simulink model "IEEE_5Bus_system_load_flow"  (R2025a)
settings: Solver=VariableStepAuto  StartTime=0.0  StopTime=10.0  RelTol=1e-3
libraries: spsThreePhasePISectionLineLib x7, spsThreePhaseVIMeasurementLib x5, spsLoadFlowBusLib x5, spsThreePhaseSeriesRLCLoadLib x4, spsThreePhaseSourceLib x2, spsThreePhaseFaultLib x1, sps_lib x1
settings Model: Creator=Hafizur Rahman  LastModifiedBy=pavan
settings RTWCC: GPUComputeCapability=3.5

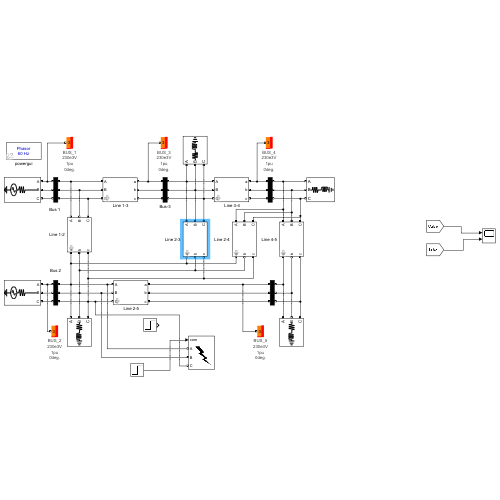
[thumbnail: Simulink's stored preview of the top-level diagram]
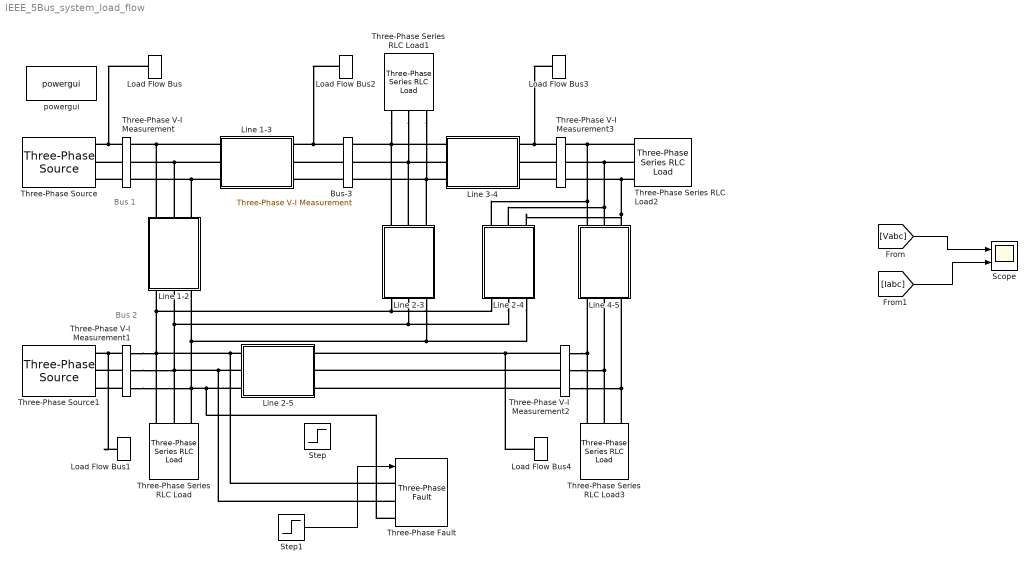
== system IEEE_5Bus_system_load_flow ==
  note: Bus 2
  note: Bus 1
  " Line 1-2" : Subsystem  mask{F=60, SB=100e6, V=230e3, R=0.02, X=0.06, B=0.06}
      mask prompts: F "Frequency"; SB "Base power"; V "Nominal Voltage"; R "Resistance(pu)"; X "Reactance(pu)"; B "Line Charging"
  " Line 1-3" : Subsystem  mask{F=60, SB=100e6, V=230e3, R=0.08, X=0.24, B=0.05}
      mask prompts: F "Frequency"; SB "Base power"; V "Nominal Voltage"; R "Resistance(pu)"; X "Reactance(pu)"; B "Line Charging"
  " Line 2-3" : Subsystem  mask{F=60, SB=100e6, V=230e3, R=0.06, X=0.18, B=0.04}
      mask prompts: F "Frequency"; SB "Base power"; V "Nominal Voltage"; R "Resistance(pu)"; X "Reactance(pu)"; B "Line Charging"
  " Line 2-4" : Subsystem  mask{F=60, SB=100e6, V=230e3, R=0.06, X=0.18, B=0.04}
      mask prompts: F "Frequency"; SB "Base power"; V "Nominal Voltage"; R "Resistance(pu)"; X "Reactance(pu)"; B "Line Charging"
  " Line 2-5" : Subsystem  mask{F=60, SB=100e6, V=230e3, R=0.04, X=0.12, B=0.03}
      mask prompts: F "Frequency"; SB "Base power"; V "Nominal Voltage"; R "Resistance(pu)"; X "Reactance(pu)"; B "Line Charging"
  " Line 3-4" : Subsystem  mask{F=60, SB=100e6, V=230e3, R=0.01, X=0.03, B=0.02}
      mask prompts: F "Frequency"; SB "Base power"; V "Nominal Voltage"; R "Resistance(pu)"; X "Reactance(pu)"; B "Line Charging"
  " Line 4-5" : Subsystem  mask{F=60, SB=100e6, V=230e3, R=0.08, X=0.24, B=0.05}
      mask prompts: F "Frequency"; SB "Base power"; V "Nominal Voltage"; R "Resistance(pu)"; X "Reactance(pu)"; B "Line Charging"
  Bus-3 : spsThreePhaseVIMeasurementLib/Three-Phase V-I Measurement  VoltageMeasurement=no  SetLabelV=off  LabelV=Vabc  Vpu=off  VpuLL=off  CurrentMeasurement=no  SetLabelI=off  LabelI=Iabc  Ipu=off  Pbase=100e6  Vbase=500e3  OutputType=Complex  PhasorSimulation=on  PSBequivalent=0
  Load Flow Bus : spsLoadFlowBusLib/Load Flow Bus  LConnTagsString=a  Phases=single  Connectors=on one side  ID=BUS_1  Vbase=230e3  Vref=1.06  Vangle=0  VLF=1  VLFb=1  VLFc=1  angleLF=0  angleLFb=0  angleLFc=0
  Load Flow Bus1 : spsLoadFlowBusLib/Load Flow Bus  LConnTagsString=a  Phases=single  Connectors=on one side  ID=BUS_2  Vbase=230e3  Vref=1  Vangle=0  VLF=1  VLFb=1  VLFc=1  angleLF=0  angleLFb=0  angleLFc=0
  Load Flow Bus2 : spsLoadFlowBusLib/Load Flow Bus  LConnTagsString=a  Phases=single  Connectors=on one side  ID=BUS_3  Vbase=230e3  Vref=1  Vangle=0  VLF=1  VLFb=1  VLFc=1  angleLF=0  angleLFb=0  angleLFc=0
  Load Flow Bus3 : spsLoadFlowBusLib/Load Flow Bus  LConnTagsString=a  Phases=single  Connectors=on one side  ID=BUS_4  Vbase=230e3  Vref=1  Vangle=0  VLF=1  VLFb=1  VLFc=1  angleLF=0  angleLFb=0  angleLFc=0
  Load Flow Bus4 : spsLoadFlowBusLib/Load Flow Bus  LConnTagsString=a  Phases=single  Connectors=on one side  ID=BUS_5  Vbase=230e3  Vref=1  Vangle=0  VLF=1  VLFb=1  VLFc=1  angleLF=0  angleLFb=0  angleLFc=0
  Scope : Scope  NumInputPorts=2
      settings: ActiveDisplayYMinimum=324868.26374899194  ActiveDisplayYMaximum=325037.04001697229
  Step : Step  SampleTime=0
  Step1 : Step  Time=5  SampleTime=0
  Three-Phase Series RLC Load : spsThreePhaseSeriesRLCLoadLib/Three-Phase Series RLC Load  LConnTagsString=A|B|C  Configuration=Y (grounded)  NominalVoltage=230e3  Vabc=[1e3 1e3 1e3]  Vabcp=[1e3 1e3 1e3]  NominalFrequency=60  UnbalancedPower=off  ActivePower=20e6  InductivePower=10e6  CapacitivePower=0  Pabc=[10e3 9e3 11e3]  QLabc=[100 90 110]  QCabc=[100 90 110]  Pabcp=[10e3 9e3 11e3]  QLabcp=[100 90 110]  QCabcp=[100 90 110]  Measurements=None  LoadType=constant PQ
  Three-Phase Series RLC Load1 : spsThreePhaseSeriesRLCLoadLib/Three-Phase Series RLC Load  LConnTagsString=A|B|C  Configuration=Y (grounded)  NominalVoltage=230e3  Vabc=[1e3 1e3 1e3]  Vabcp=[1e3 1e3 1e3]  NominalFrequency=60  UnbalancedPower=off  ActivePower=45e6  InductivePower=15e6  CapacitivePower=0  Pabc=[10e3 9e3 11e3]  QLabc=[100 90 110]  QCabc=[100 90 110]  Pabcp=[10e3 9e3 11e3]  QLabcp=[100 90 110]  QCabcp=[100 90 110]  Measurements=None  LoadType=constant PQ
  Three-Phase Series RLC Load2 : spsThreePhaseSeriesRLCLoadLib/Three-Phase Series RLC Load  LConnTagsString=A|B|C  Configuration=Y (grounded)  NominalVoltage=230e3  Vabc=[1e3 1e3 1e3]  Vabcp=[1e3 1e3 1e3]  NominalFrequency=60  UnbalancedPower=off  ActivePower=40e6  InductivePower=5e6  CapacitivePower=0  Pabc=[10e3 9e3 11e3]  QLabc=[100 90 110]  QCabc=[100 90 110]  Pabcp=[10e3 9e3 11e3]  QLabcp=[100 90 110]  QCabcp=[100 90 110]  Measurements=None  LoadType=constant PQ
  Three-Phase Series RLC Load3 : spsThreePhaseSeriesRLCLoadLib/Three-Phase Series RLC Load  LConnTagsString=A|B|C  Configuration=Y (grounded)  NominalVoltage=230e3  Vabc=[1e3 1e3 1e3]  Vabcp=[1e3 1e3 1e3]  NominalFrequency=60  UnbalancedPower=off  ActivePower=60e6  InductivePower=10e6  CapacitivePower=0  Pabc=[10e3 9e3 11e3]  QLabc=[100 90 110]  QCabc=[100 90 110]  Pabcp=[10e3 9e3 11e3]  QLabcp=[100 90 110]  QCabcp=[100 90 110]  Measurements=None  LoadType=constant PQ
  Three-Phase V-I Measurement : spsThreePhaseVIMeasurementLib/Three-Phase V-I Measurement  VoltageMeasurement=no  SetLabelV=off  LabelV=Vabc  Vpu=off  VpuLL=off  CurrentMeasurement=no  SetLabelI=off  LabelI=Iabc  Ipu=off  Pbase=100e6  Vbase=500e3  OutputType=Complex  PhasorSimulation=on  PSBequivalent=0
  Three-Phase V-I Measurement1 : spsThreePhaseVIMeasurementLib/Three-Phase V-I Measurement  VoltageMeasurement=phase-to-phase  SetLabelV=on  LabelV=Vabc  Vpu=off  VpuLL=off  CurrentMeasurement=yes  SetLabelI=on  LabelI=Iabc  Ipu=off  Pbase=100e6  Vbase=500e3  OutputType=Magnitude  PhasorSimulation=on  PSBequivalent=0
  Three-Phase V-I Measurement2 : spsThreePhaseVIMeasurementLib/Three-Phase V-I Measurement  VoltageMeasurement=no  SetLabelV=off  LabelV=Vabc  Vpu=off  VpuLL=off  CurrentMeasurement=no  SetLabelI=off  LabelI=Iabc  Ipu=off  Pbase=100e6  Vbase=500e3  OutputType=Complex  PhasorSimulation=on  PSBequivalent=0
  Three-Phase V-I Measurement3 : spsThreePhaseVIMeasurementLib/Three-Phase V-I Measurement  VoltageMeasurement=no  SetLabelV=off  LabelV=Vabc  Vpu=off  VpuLL=off  CurrentMeasurement=no  SetLabelI=off  LabelI=Iabc  Ipu=off  Pbase=100e6  Vbase=500e3  OutputType=Complex  PhasorSimulation=on  PSBequivalent=0
  Three-Phase Fault : spsThreePhaseFaultLib/Three-Phase Fault  InitialStates=0  FaultA=on  FaultB=on  FaultC=on  GroundFault=on  SwitchTimes="[1/60  5/60]"  External=on  SwitchStatus=NaN  FaultResistance=0.001  GroundResistance=0.01  SnubberResistance=1e6  SnubberCapacitance=inf  Measurements=None
  Three-Phase Source : spsThreePhaseSourceLib/Three-Phase Source  InternalConnection=Yg  VoltagePhases=off  Voltage=1.06*230e3  PhaseAngle=0  Voltage_phases=[25e3 25e3 25e3]/sqrt(3)  PhaseAngles_phases=[0 -120 +120]  Frequency=60  NonIdealSource=on  SpecifyImpedance=off  Resistance=1e-6  Inductance=0  ShortCircuitLevel=100e6  BaseVoltage=230e3  XRratio=7  BusType=swing  Pref=10e3  Qref=0  Prefabc=[10e3, 10e3, 10e3]  Qrefabc=[0, 0, 0]  Qmin=-inf  Qmax=inf
  Three-Phase Source1 : spsThreePhaseSourceLib/Three-Phase Source  InternalConnection=Yg  VoltagePhases=off  Voltage=230e3  PhaseAngle=0  Voltage_phases=[25e3 25e3 25e3]/sqrt(3)  PhaseAngles_phases=[0 -120 +120]  Frequency=60  NonIdealSource=on  SpecifyImpedance=off  Resistance=1e-6  Inductance=0  ShortCircuitLevel=100e6  BaseVoltage=230e3  XRratio=7  BusType=PV  Pref=40e6  Qref=0  Prefabc=[10e3, 10e3, 10e3]  Qrefabc=[0, 0, 0]  Qmin=-300e6  Qmax=300e6
  powergui : sps_lib/powergui  Priority=1  SimulationMode=Phasor  SampleTime=50e-6  frequency=60  Iterations=50  frequencyindice=60  Pbase=100e6  ErrMax=1e-4  UnitsV=kV  UnitsW=MW  buscounter=0  FunctionMessages=off  echomessages=off  EnableUseOfTLC=off  CurrentSourceSwitches=off  DisableSnubberDevices=off  DisableRonSwitches=off  DisableVfSwitches=off  DisplayEquations=off  AutomaticDiscreteSolvers=off  SolverType=Tustin/Backward Euler (TBE)  Interpol=off  ExternalGateDelay=off  methode=off  Ts=100  x0status=blocks  SPID=on  SwTol=0  HookPort=off  NonlinearTolerance=1e-4  nMaxIteration=100  ContinueOnMaxIteration=off  RestoreLinks=warning  ResistiveCurrentMeasurement=off  Frange=[0:2:500]  Ylog=off  Xlog=on  ShowGrid=off  save=off  variable=ZData  structure=0  ZoomFFT=off  StartTime=0.0  cycles=1  DisplayStyle=1  fundamental=60  FreqAxis=off  MaxFrequency=1000  frequencyindicesteady=1  RmsSteady=1  display=off
  wires:
  Step1/1 -> Three-Phase Fault/1
  [Vabc] -> Scope/1
  [Iabc] -> Scope/2
  connections:
  Three-Phase V-I Measurement/LConn2 -- Three-Phase Source/RConn2
  Three-Phase V-I Measurement/LConn1 -- Load Flow Bus/LConn1 -- Three-Phase Source/RConn1
  Three-Phase V-I Measurement/LConn3 -- Three-Phase Source/RConn3
  " Line 1-3"/LConn1 -- " Line 1-2"/LConn1 -- Three-Phase V-I Measurement/RConn1
  " Line 1-3"/LConn2 -- " Line 1-2"/LConn2 -- Three-Phase V-I Measurement/RConn2
  " Line 1-3"/LConn3 -- " Line 1-2"/LConn3 -- Three-Phase V-I Measurement/RConn3
  Three-Phase V-I Measurement1/LConn1 -- Load Flow Bus1/LConn1 -- Three-Phase Source1/RConn1
  Three-Phase V-I Measurement1/LConn2 -- Three-Phase Source1/RConn2
  Three-Phase V-I Measurement1/LConn3 -- Three-Phase Source1/RConn3
  Three-Phase V-I Measurement1/RConn1 -- Three-Phase Fault/LConn1 -- " Line 2-5"/LConn1 -- Three-Phase Series RLC Load/LConn1 -- " Line 2-4"/RConn1 -- " Line 2-3"/RConn1 -- " Line 1-2"/RConn1
  Three-Phase V-I Measurement1/RConn2 -- Three-Phase Fault/LConn2 -- " Line 2-5"/LConn2 -- Three-Phase Series RLC Load/LConn2 -- " Line 2-4"/RConn2 -- " Line 2-3"/RConn2 -- " Line 1-2"/RConn2
  Three-Phase V-I Measurement1/RConn3 -- Three-Phase Fault/LConn3 -- " Line 2-5"/LConn3 -- Three-Phase Series RLC Load/LConn3 -- " Line 2-4"/RConn3 -- " Line 2-3"/RConn3 -- " Line 1-2"/RConn3
  Bus-3/LConn1 -- Load Flow Bus2/LConn1 -- " Line 1-3"/RConn1
  Bus-3/LConn2 -- " Line 1-3"/RConn2
  Bus-3/LConn3 -- " Line 1-3"/RConn3
  " Line 3-4"/LConn1 -- " Line 2-3"/LConn1 -- Three-Phase Series RLC Load1/LConn1 -- Bus-3/RConn1
  " Line 3-4"/LConn2 -- " Line 2-3"/LConn2 -- Three-Phase Series RLC Load1/LConn2 -- Bus-3/RConn2
  " Line 3-4"/LConn3 -- " Line 2-3"/LConn3 -- Three-Phase Series RLC Load1/LConn3 -- Bus-3/RConn3
  Three-Phase V-I Measurement3/LConn1 -- Load Flow Bus3/LConn1 -- " Line 3-4"/RConn1
  Three-Phase V-I Measurement3/LConn2 -- " Line 3-4"/RConn2
  Three-Phase V-I Measurement3/LConn3 -- " Line 3-4"/RConn3
  Three-Phase Series RLC Load2/LConn1 -- " Line 4-5"/LConn1 -- " Line 2-4"/LConn1 -- Three-Phase V-I Measurement3/RConn1
  Three-Phase Series RLC Load2/LConn2 -- " Line 2-4"/LConn2 -- " Line 4-5"/LConn2 -- Three-Phase V-I Measurement3/RConn2
  Three-Phase Series RLC Load2/LConn3 -- " Line 2-4"/LConn3 -- " Line 4-5"/LConn3 -- Three-Phase V-I Measurement3/RConn3
  Three-Phase V-I Measurement2/LConn1 -- Load Flow Bus4/LConn1 -- " Line 2-5"/RConn1
  Three-Phase V-I Measurement2/LConn3 -- " Line 2-5"/RConn3
  Three-Phase V-I Measurement2/RConn1 -- Three-Phase Series RLC Load3/LConn1 -- " Line 4-5"/RConn1
  Three-Phase V-I Measurement2/RConn2 -- Three-Phase Series RLC Load3/LConn2 -- " Line 4-5"/RConn2
  Three-Phase V-I Measurement2/RConn3 -- Three-Phase Series RLC Load3/LConn3 -- " Line 4-5"/RConn3
  Three-Phase V-I Measurement2/LConn2 -- " Line 2-5"/RConn2

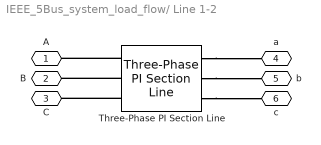
== system IEEE_5Bus_system_load_flow/ Line 1-2 ==
  Three-Phase PI Section Line : spsThreePhasePISectionLineLib/Three-Phase PI Section Line  LConnTagsString=a|b|c  RConnTagsString=A|B|C  Length=floor((3e5)*(sqrt(X*B))/(2*pi*F))  Frequency=F  Resistances=[ (R*(V^2)/SB)/floor((3e5)*(sqrt(X*B))/(2*pi*F)) 3*(R*(V^2)/SB)/floor((3e5)*(sqrt(X*B))/(2*pi*F))]  Inductances=[ (X*(V^2)/SB)/(2*pi*F*floor((3e5)*(sqrt(X*B))/(2*pi*F))) 3*(X*(V^2)/SB)/(2*pi*F*floor((3e5)*(sqrt(X*B))/(2*pi*F)))]  Capacitances=[(B*SB)/((floor((3e5)*(sqrt(X*B))/(2*pi*F)))*2*pi*F*V^2) (3*B*SB)/((floor((3e5)*(sqrt(X*B))/(2*pi*F)))*2*pi*F*V^2)]
  A : PMIOPort  Side=Left
  B : PMIOPort  Port=2  Side=Left
  C : PMIOPort  Port=3  Side=Left
  a : PMIOPort  Port=4  Side=Right
  b : PMIOPort  Port=5  Side=Right
  c : PMIOPort  Port=6  Side=Right
  connections:
  Three-Phase PI Section Line/RConn1 -- a/RConn1
  Three-Phase PI Section Line/LConn3 -- C/RConn1
  Three-Phase PI Section Line/LConn1 -- A/RConn1
  Three-Phase PI Section Line/RConn3 -- c/RConn1
  Three-Phase PI Section Line/RConn2 -- b/RConn1
  Three-Phase PI Section Line/LConn2 -- B/RConn1

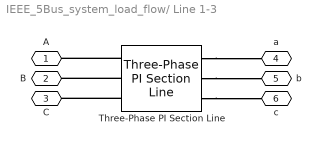
== system IEEE_5Bus_system_load_flow/ Line 1-3 ==
  Three-Phase PI Section Line : spsThreePhasePISectionLineLib/Three-Phase PI Section Line  LConnTagsString=a|b|c  RConnTagsString=A|B|C  Length=floor((3e5)*(sqrt(X*B))/(2*pi*F))  Frequency=F  Resistances=[ (R*(V^2)/SB)/floor((3e5)*(sqrt(X*B))/(2*pi*F)) 3*(R*(V^2)/SB)/floor((3e5)*(sqrt(X*B))/(2*pi*F))]  Inductances=[ (X*(V^2)/SB)/(2*pi*F*floor((3e5)*(sqrt(X*B))/(2*pi*F))) 3*(X*(V^2)/SB)/(2*pi*F*floor((3e5)*(sqrt(X*B))/(2*pi*F)))]  Capacitances=[(B*SB)/((floor((3e5)*(sqrt(X*B))/(2*pi*F)))*2*pi*F*V^2) (3*B*SB)/((floor((3e5)*(sqrt(X*B))/(2*pi*F)))*2*pi*F*V^2)]
  A : PMIOPort  Side=Left
  B : PMIOPort  Port=2  Side=Left
  C : PMIOPort  Port=3  Side=Left
  a : PMIOPort  Port=4  Side=Right
  b : PMIOPort  Port=5  Side=Right
  c : PMIOPort  Port=6  Side=Right
  connections:
  Three-Phase PI Section Line/LConn2 -- B/RConn1
  Three-Phase PI Section Line/RConn2 -- b/RConn1
  Three-Phase PI Section Line/RConn3 -- c/RConn1
  Three-Phase PI Section Line/LConn1 -- A/RConn1
  Three-Phase PI Section Line/LConn3 -- C/RConn1
  Three-Phase PI Section Line/RConn1 -- a/RConn1

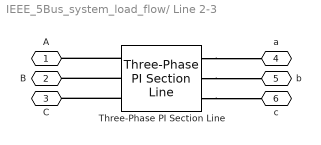
== system IEEE_5Bus_system_load_flow/ Line 2-3 ==
  Three-Phase PI Section Line : spsThreePhasePISectionLineLib/Three-Phase PI Section Line  LConnTagsString=a|b|c  RConnTagsString=A|B|C  Length=floor((3e5)*(sqrt(X*B))/(2*pi*F))  Frequency=F  Resistances=[ (R*(V^2)/SB)/floor((3e5)*(sqrt(X*B))/(2*pi*F)) 3*(R*(V^2)/SB)/floor((3e5)*(sqrt(X*B))/(2*pi*F))]  Inductances=[ (X*(V^2)/SB)/(2*pi*F*floor((3e5)*(sqrt(X*B))/(2*pi*F))) 3*(X*(V^2)/SB)/(2*pi*F*floor((3e5)*(sqrt(X*B))/(2*pi*F)))]  Capacitances=[(B*SB)/((floor((3e5)*(sqrt(X*B))/(2*pi*F)))*2*pi*F*V^2) (3*B*SB)/((floor((3e5)*(sqrt(X*B))/(2*pi*F)))*2*pi*F*V^2)]
  A : PMIOPort  Side=Left
  B : PMIOPort  Port=2  Side=Left
  C : PMIOPort  Port=3  Side=Left
  a : PMIOPort  Port=4  Side=Right
  b : PMIOPort  Port=5  Side=Right
  c : PMIOPort  Port=6  Side=Right
  connections:
  Three-Phase PI Section Line/LConn2 -- B/RConn1
  Three-Phase PI Section Line/RConn2 -- b/RConn1
  Three-Phase PI Section Line/RConn3 -- c/RConn1
  Three-Phase PI Section Line/LConn1 -- A/RConn1
  Three-Phase PI Section Line/LConn3 -- C/RConn1
  Three-Phase PI Section Line/RConn1 -- a/RConn1

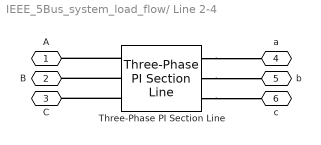
== system IEEE_5Bus_system_load_flow/ Line 2-4 ==
  Three-Phase PI Section Line : spsThreePhasePISectionLineLib/Three-Phase PI Section Line  LConnTagsString=a|b|c  RConnTagsString=A|B|C  Length=floor((3e5)*(sqrt(X*B))/(2*pi*F))  Frequency=F  Resistances=[ (R*(V^2)/SB)/floor((3e5)*(sqrt(X*B))/(2*pi*F)) 3*(R*(V^2)/SB)/floor((3e5)*(sqrt(X*B))/(2*pi*F))]  Inductances=[ (X*(V^2)/SB)/(2*pi*F*floor((3e5)*(sqrt(X*B))/(2*pi*F))) 3*(X*(V^2)/SB)/(2*pi*F*floor((3e5)*(sqrt(X*B))/(2*pi*F)))]  Capacitances=[(B*SB)/((floor((3e5)*(sqrt(X*B))/(2*pi*F)))*2*pi*F*V^2) (3*B*SB)/((floor((3e5)*(sqrt(X*B))/(2*pi*F)))*2*pi*F*V^2)]
  A : PMIOPort  Side=Left
  B : PMIOPort  Port=2  Side=Left
  C : PMIOPort  Port=3  Side=Left
  a : PMIOPort  Port=4  Side=Right
  b : PMIOPort  Port=5  Side=Right
  c : PMIOPort  Port=6  Side=Right
  connections:
  Three-Phase PI Section Line/RConn1 -- a/RConn1
  Three-Phase PI Section Line/LConn3 -- C/RConn1
  Three-Phase PI Section Line/LConn1 -- A/RConn1
  Three-Phase PI Section Line/RConn3 -- c/RConn1
  Three-Phase PI Section Line/RConn2 -- b/RConn1
  Three-Phase PI Section Line/LConn2 -- B/RConn1

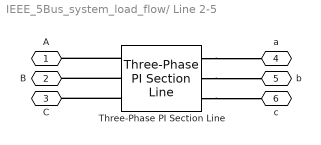
== system IEEE_5Bus_system_load_flow/ Line 2-5 ==
  Three-Phase PI Section Line : spsThreePhasePISectionLineLib/Three-Phase PI Section Line  LConnTagsString=a|b|c  RConnTagsString=A|B|C  Length=floor((3e5)*(sqrt(X*B))/(2*pi*F))  Frequency=F  Resistances=[ (R*(V^2)/SB)/floor((3e5)*(sqrt(X*B))/(2*pi*F)) 3*(R*(V^2)/SB)/floor((3e5)*(sqrt(X*B))/(2*pi*F))]  Inductances=[ (X*(V^2)/SB)/(2*pi*F*floor((3e5)*(sqrt(X*B))/(2*pi*F))) 3*(X*(V^2)/SB)/(2*pi*F*floor((3e5)*(sqrt(X*B))/(2*pi*F)))]  Capacitances=[(B*SB)/((floor((3e5)*(sqrt(X*B))/(2*pi*F)))*2*pi*F*V^2) (3*B*SB)/((floor((3e5)*(sqrt(X*B))/(2*pi*F)))*2*pi*F*V^2)]
  A : PMIOPort  Side=Left
  B : PMIOPort  Port=2  Side=Left
  C : PMIOPort  Port=3  Side=Left
  a : PMIOPort  Port=4  Side=Right
  b : PMIOPort  Port=5  Side=Right
  c : PMIOPort  Port=6  Side=Right
  connections:
  Three-Phase PI Section Line/LConn2 -- B/RConn1
  Three-Phase PI Section Line/RConn2 -- b/RConn1
  Three-Phase PI Section Line/RConn3 -- c/RConn1
  Three-Phase PI Section Line/LConn1 -- A/RConn1
  Three-Phase PI Section Line/LConn3 -- C/RConn1
  Three-Phase PI Section Line/RConn1 -- a/RConn1

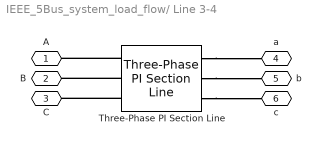
== system IEEE_5Bus_system_load_flow/ Line 3-4 ==
  Three-Phase PI Section Line : spsThreePhasePISectionLineLib/Three-Phase PI Section Line  LConnTagsString=a|b|c  RConnTagsString=A|B|C  Length=floor((3e5)*(sqrt(X*B))/(2*pi*F))  Frequency=F  Resistances=[ (R*(V^2)/SB)/floor((3e5)*(sqrt(X*B))/(2*pi*F)) 3*(R*(V^2)/SB)/floor((3e5)*(sqrt(X*B))/(2*pi*F))]  Inductances=[ (X*(V^2)/SB)/(2*pi*F*floor((3e5)*(sqrt(X*B))/(2*pi*F))) 3*(X*(V^2)/SB)/(2*pi*F*floor((3e5)*(sqrt(X*B))/(2*pi*F)))]  Capacitances=[(B*SB)/((floor((3e5)*(sqrt(X*B))/(2*pi*F)))*2*pi*F*V^2) (3*B*SB)/((floor((3e5)*(sqrt(X*B))/(2*pi*F)))*2*pi*F*V^2)]
  A : PMIOPort  Side=Left
  B : PMIOPort  Port=2  Side=Left
  C : PMIOPort  Port=3  Side=Left
  a : PMIOPort  Port=4  Side=Right
  b : PMIOPort  Port=5  Side=Right
  c : PMIOPort  Port=6  Side=Right
  connections:
  Three-Phase PI Section Line/RConn1 -- a/RConn1
  Three-Phase PI Section Line/LConn3 -- C/RConn1
  Three-Phase PI Section Line/LConn1 -- A/RConn1
  Three-Phase PI Section Line/RConn3 -- c/RConn1
  Three-Phase PI Section Line/RConn2 -- b/RConn1
  Three-Phase PI Section Line/LConn2 -- B/RConn1

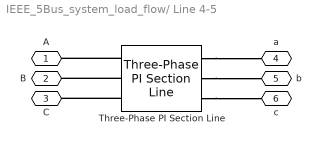
== system IEEE_5Bus_system_load_flow/ Line 4-5 ==
  Three-Phase PI Section Line : spsThreePhasePISectionLineLib/Three-Phase PI Section Line  LConnTagsString=a|b|c  RConnTagsString=A|B|C  Length=floor((3e5)*(sqrt(X*B))/(2*pi*F))  Frequency=F  Resistances=[ (R*(V^2)/SB)/floor((3e5)*(sqrt(X*B))/(2*pi*F)) 3*(R*(V^2)/SB)/floor((3e5)*(sqrt(X*B))/(2*pi*F))]  Inductances=[ (X*(V^2)/SB)/(2*pi*F*floor((3e5)*(sqrt(X*B))/(2*pi*F))) 3*(X*(V^2)/SB)/(2*pi*F*floor((3e5)*(sqrt(X*B))/(2*pi*F)))]  Capacitances=[(B*SB)/((floor((3e5)*(sqrt(X*B))/(2*pi*F)))*2*pi*F*V^2) (3*B*SB)/((floor((3e5)*(sqrt(X*B))/(2*pi*F)))*2*pi*F*V^2)]
  A : PMIOPort  Side=Left
  B : PMIOPort  Port=2  Side=Left
  C : PMIOPort  Port=3  Side=Left
  a : PMIOPort  Port=4  Side=Right
  b : PMIOPort  Port=5  Side=Right
  c : PMIOPort  Port=6  Side=Right
  connections:
  Three-Phase PI Section Line/LConn2 -- B/RConn1
  Three-Phase PI Section Line/RConn2 -- b/RConn1
  Three-Phase PI Section Line/RConn3 -- c/RConn1
  Three-Phase PI Section Line/LConn1 -- A/RConn1
  Three-Phase PI Section Line/LConn3 -- C/RConn1
  Three-Phase PI Section Line/RConn1 -- a/RConn1
